simulink model "wahadlo"  (R2022b)
settings: Solver=ode45  StartTime=0.0  StopTime=simulation_time  FixedStep=0.05  RelTol=1e-5  AbsTol=1e-6
PreLoadFcn:
  | theta1_ddot=0;
  | theta2_ddot=0;
model workspace (MAT data in the model file):
  epsilon = 1
  pend = [0.036 0 0.05 0.1 0.022 0.05 0.045 0.015 -0.005 -5e-05 9.81 4.356e-05 5e-05 8.106e-05]
  simulation_step = 0.025
  simulation_time = 25
  theta0 = 0
  theta1 = 0
  theta10 = 0
  theta10_dot = 10
  theta1_dot = 0
  theta2 = 0
  theta20 = 0
  theta20_dot = 0
  theta2_dot = 0
  theta_dot = 0
undefined symbols (not defined in the file): a, opts, tau2
libraries: vrlib x1
settings Model: Creator=Paweł Zieliński  LastModifiedBy=norma
settings SolverCC: AutoScaleAbsTol=off  AlgebraicLoopSolver=TrustRegion  DecoupledContinuousIntegration=on  MinimalZcImpactIntegration=on
settings DataIOCC: SignalLogging=off
settings DebuggingCC: UnconnectedInputMsg=warning  UnconnectedOutputMsg=warning  UnconnectedLineMsg=warning  SFMachineParentedDataDiag=warning
settings ModelReferenceCC: EnableRefExpFcnMdlSchedulingChecks=on
settings RTWCC: DLArmComputeVersion=19.05

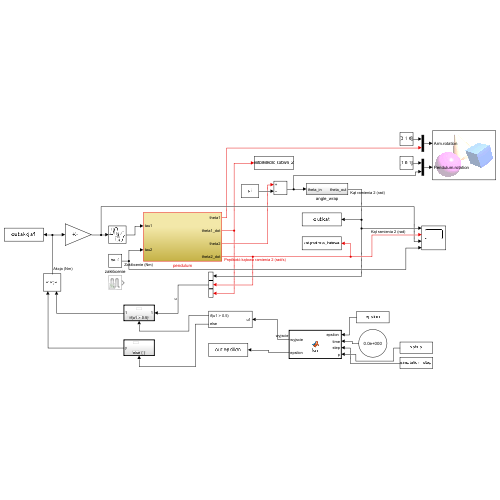
[thumbnail: Simulink's stored preview of the top-level diagram]
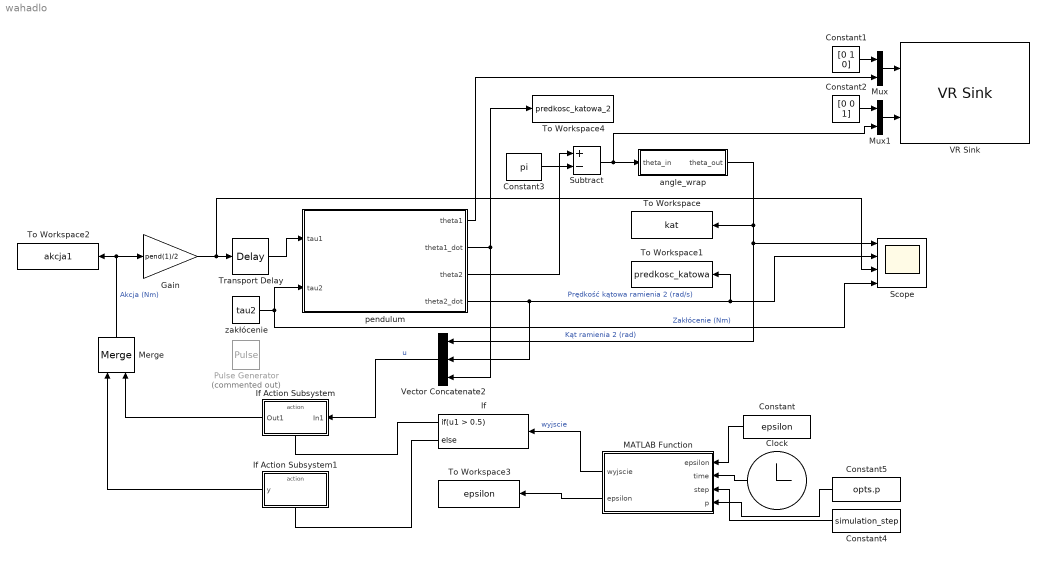
== system wahadlo ==
  Clock : Clock
  Constant : Constant  Value=epsilon  SampleTime=simulation_step
  Constant1 : Constant  Value=[0 1 0]
  Constant2 : Constant  Value=[0 0 1]
  Constant3 : Constant  Value=pi
  Constant4 : Constant  Value=simulation_step  SampleTime=simulation_step
  Constant5 : Constant  Value=opts.p  SampleTime=simulation_step
  Gain : Gain  Gain=pend(1)/2
  If : If  IfExpression=u1 > 0.5
  If Action Subsystem : Subsystem  TreatAsAtomicUnit=on
  If Action Subsystem1 : Subsystem  TreatAsAtomicUnit=on
  MATLAB Function : MATLAB Function  TreatAsAtomicUnit=on  SystemSampleTime=0.025
  Merge : Merge
  Mux : Mux  Inputs=2
  Mux1 : Mux  Inputs=2
  Pulse Generator : DiscretePulseGenerator  Commented=on  PulseType=Time based  Amplitude=0.066  Period=5  PulseWidth=0.05  PhaseDelay=5
  Scope : Scope  NumInputPorts=4
  Subtract : Sum  Inputs=+-
  To Workspace : ToWorkspace  VariableName=kat  SampleTime=simulation_step
  To Workspace1 : ToWorkspace  VariableName=predkosc_katowa  SampleTime=simulation_step
  To Workspace2 : ToWorkspace  VariableName=akcja1  SampleTime=simulation_step
  To Workspace3 : ToWorkspace  VariableName=epsilon  SampleTime=simulation_step
  To Workspace4 : ToWorkspace  VariableName=predkosc_katowa_2  SampleTime=simulation_step
  Transport Delay : TransportDelay  DelayTime=opts.t_delay
  VR Sink : vrlib/VR Sink  InstantiateOnLoad=on  SampleTime=0.02  ViewEnable=on  RemoteChange=off  RemoteView=off  FieldsWritten=Arm.rotation.4.1.1.double#Pendulum.rotation.4.1.1.double  WorldFileName=Furut.x3d  AutoView=on  VideoDimensions=[]  AllowVariableSize=off  FigureProperties="{'Position', 'Name', 'Viewpoint', 'CameraBound', 'CameraDirection', 'CameraPosition', 'CameraUpVector', 'ZoomFactor', 'Antialiasing', 'Headlight', 'Lighting', 'NavPanel', 'Sound', 'StatusBar', 'Stereo3D', 'Stereo3DCameraOffset', 'Stereo3DHIT', 'ToolBar', 'Textures', 'Transparency', 'Triad', 'Wireframe', 'NavZones', 'NavMode', 'NavSpeed', 'CaptureFileFormat', 'CaptureFileName', 'Record2DCompressMethod', 'Record2DCompressQuality', 'Record2D', 'Record2DFileName', 'Record2DFPS'; [1.8180000000000001e+02   3.5100000000000000e+02   5.7600000000000000e+02   3.5000000000000000e+02], '', '', 'on', [-6.0993984428009929e-01  -2.4882720041061857e-01  -7.5236853382859903e-01], [5.4254469456383454e+00   3.1603074248017142e+00   6.5087241804420986e+00], [-6.1950849615539330e-02   9.6149025744211092e-01  -2.6776589976286658e-01], [1.0000000000000000e+00], 'on', 'on', 'on', 'halfbar', 'on', 'on', 'off', [1.0000000149011612e-01], [0.0000000000000000e+00], 'on', 'on', 'on', 'none', 'off', 'off', 'examine', 'normal', 'tif', '%f_anim_%n.tif', 'auto', [7.5000000000000000e+01], 'off', '%f_anim_%n.avi', 'auto'}"
  Vector Concatenate2 : Concatenate  NumInputs=3
  angle_wrap : Subsystem
  pendulum : Subsystem
  zakłócenie : Constant  Value=tau2
  wires:
  angle_wrap/1(theta_out) -> Vector Concatenate2/1, Scope/1, To Workspace/1  "Kąt ramienia 2 (rad)"
  Constant/1 -> MATLAB Function/1("epsilon ")
  Clock/1 -> MATLAB Function/2(time)
  MATLAB Function/2(epsilon) -> To Workspace3/1
  Vector Concatenate2/1 -> If Action Subsystem/1(In1)  "u"
  MATLAB Function/1(wyjscie) -> If/1  "wyjscie"
  If/1 -> If Action Subsystem/Action
  If/2 -> If Action Subsystem1/Action
  If Action Subsystem1/1(y) -> Merge/1
  If Action Subsystem/1(Out1) -> Merge/2
  Constant1/1 -> Mux/1
  Constant2/1 -> Mux1/1
  pendulum/3(theta2) -> Subtract/1
  Mux/1 -> VR Sink/1
  Mux1/1 -> VR Sink/2
  Constant3/1 -> Subtract/2
  Merge/1 -> Gain/1, To Workspace2/1  "Akcja (Nm)"
  pendulum/4(theta2_dot) -> Vector Concatenate2/2, To Workspace1/1, Scope/2  "Prędkość kątowa ramienia 2 (rad/s)"
  pendulum/2(theta1_dot) -> To Workspace4/1, Vector Concatenate2/3
  Constant4/1 -> MATLAB Function/3(step)
  pendulum/1(theta1) -> Mux/2
  Subtract/1 -> Mux1/2, angle_wrap/1(theta_in)
  Transport Delay/1 -> pendulum/1(tau1)
  Gain/1 -> Scope/3, Transport Delay/1
  zakłócenie/1 -> pendulum/2(tau2), Scope/4  "Zakłócenie (Nm)"
  Constant5/1 -> MATLAB Function/4(p)

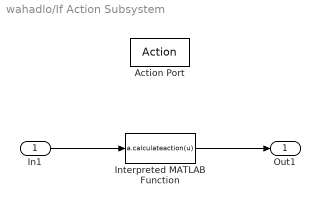
== system wahadlo/If Action Subsystem ==
  In1 : Inport  SampleTime=simulation_step
  Action Port : ActionPort  ActionPortLabel=if(u1 > 0.5)
  Interpreted MATLAB Function : MATLABFcn  MATLABFcn=a.calculateaction(u)
  Out1 : Outport  SampleTime=simulation_step
  wires:
  In1/1 -> Interpreted MATLAB Function/1
  Interpreted MATLAB Function/1 -> Out1/1

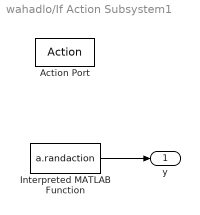
== system wahadlo/If Action Subsystem1 ==
  Action Port : ActionPort  ActionPortLabel=else
  Interpreted MATLAB Function : MATLABFcn  MATLABFcn=a.randaction
  y : Outport  SampleTime=simulation_step
  wires:
  Interpreted MATLAB Function/1 -> y/1

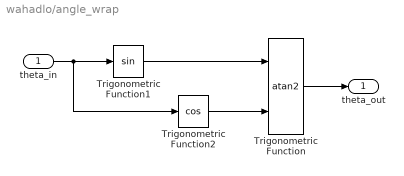
== system wahadlo/angle_wrap ==
  theta_in : Inport  SampleTime=simulation_step
  Trigonometric Function : Trigonometry  Operator=atan2
  Trigonometric Function1 : Trigonometry
  Trigonometric Function2 : Trigonometry  Operator=cos
  theta_out : Outport  SampleTime=simulation_step  VectorParamsAs1DForOutWhenUnconnected=off
  wires:
  theta_in/1 -> Trigonometric Function2/1, Trigonometric Function1/1
  Trigonometric Function/1 -> theta_out/1
  Trigonometric Function1/1 -> Trigonometric Function/1
  Trigonometric Function2/1 -> Trigonometric Function/2

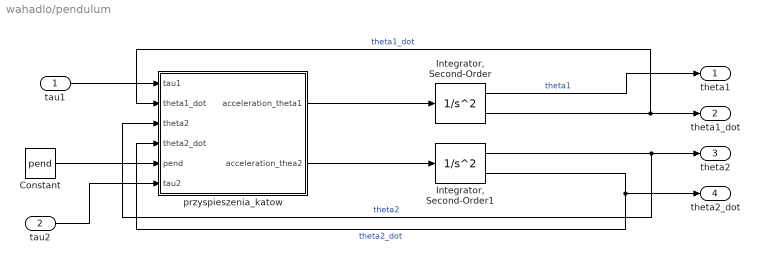
== system wahadlo/pendulum ==
  tau1 : Inport
  tau2 : Inport  Port=2
  Constant : Constant  Value=pend  SampleTime=1
  "Integrator, Second-Order" : SecondOrderIntegrator  ICX=theta10  UpperLimitX=1  LowerLimitX=0  WrapX=on  WrappedUpperValueX=2*pi  WrappedLowerValueX=0  StateNameX='theta1'  ICDXDT=theta10_dot  LimitDXDT=on  UpperLimitDXDT=20  LowerLimitDXDT=-20  StateNameDXDT='theta1_dot'
  "Integrator, Second-Order1" : SecondOrderIntegrator  ICX=theta20  UpperLimitX=1  LowerLimitX=0  WrapX=on  WrappedUpperValueX=2*pi  WrappedLowerValueX=0  StateNameX='theta2'  ICDXDT=theta20_dot  LimitDXDT=on  UpperLimitDXDT=40  LowerLimitDXDT=-40  StateNameDXDT='theta2_dot'
  przyspieszenia_katow : MATLAB Function  TreatAsAtomicUnit=on  SystemSampleTime=0.0
  theta1 : Outport  VectorParamsAs1DForOutWhenUnconnected=off
  theta1_dot : Outport  Port=2  VectorParamsAs1DForOutWhenUnconnected=off
  theta2 : Outport  Port=3  VectorParamsAs1DForOutWhenUnconnected=off
  theta2_dot : Outport  Port=4  VectorParamsAs1DForOutWhenUnconnected=off
  wires:
  "Integrator, Second-Order"/1 -> theta1/1  "theta1"
  przyspieszenia_katow/1(acceleration_theta1) -> "Integrator, Second-Order"/1
  "Integrator, Second-Order"/2 -> przyspieszenia_katow/2(theta1_dot), theta1_dot/1  "theta1_dot"
  przyspieszenia_katow/2(acceleration_thea2) -> "Integrator, Second-Order1"/1
  "Integrator, Second-Order1"/1 -> przyspieszenia_katow/3(theta2), theta2/1  "theta2"
  "Integrator, Second-Order1"/2 -> przyspieszenia_katow/4(theta2_dot), theta2_dot/1  "theta2_dot"
  Constant/1 -> przyspieszenia_katow/5(pend)
  tau1/1 -> przyspieszenia_katow/1(tau1)
  tau2/1 -> przyspieszenia_katow/6(tau2)

== matlab function wahadlo/MATLAB Function ==
  data: epsilon input; wyjscie output; time input; step input; epsilon output; p input
function [wyjscie,epsilon] = fcn(epsilon,time,step,p)

if(epsilon>=0.02)
epsilon = max(epsilon*(p)^(time/step), 0.02);
else
epsilon=epsilon;
end

if (unifrnd(0, 1) < epsilon)
    wyjscie=0;
else
    wyjscie=1;  
end

== matlab function wahadlo/pendulum/przyspieszenia_katow ==
  data: tau1 input; acceleration_theta1 output; theta1_dot input; theta2 input; theta2_dot input; acceleration_thea2 output; pend input; tau2 input
function [acceleration_theta1,acceleration_thea2] = fcn1(tau1,theta1_dot, theta2, theta2_dot,pend,tau2)

pend(2)=tau2;

X = [pend(14)+pend(13)*(sin(theta2))^2 pend(8)*pend(3)*pend(6)*cos(theta2);pend(8)*pend(3)*pend(6)*cos(theta2) pend(13)]^(-1) * ...
    ([pend(9)+0.5*theta2_dot*pend(13)*sin(2*theta2) 0.5*theta2_dot*pend(13)*sin(2*theta2) ...
    - pend(8)*pend(3)*pend(6)*sin(theta2)*theta2_dot; -0.5*theta1_dot*pend(13)*sin(2*theta2) pend(10)]* ...
    [theta1_dot;theta2_dot]-[0;pend(11)*pend(8)*pend(6)*sin(theta2)]+[tau1;tau2]);

acceleration_theta1=X(1,1);
acceleration_thea2=X(2,1);
